simulink model "kalman_filter"  (R2020b)
settings: Solver=ode1  StartTime=0.0  StopTime=30  FixedStep=0.002  RelTol=1e-3  EnableMultiTasking=on
PreLoadFcn:
  | quanser_aero_lqr
undefined symbols (not defined in the file or in its folder): HIL, qc_get_step_size
libraries: quarc_library x4
settings Model: SimulationMode=external  ExtModeTrigDuration=20000  Creator=MLevis  LastModifiedBy=ffsandva
settings SolverCC: PositivePriorityOrder=on
settings DataIOCC: LimitDataPoints=on  SaveFormat=Array  ReturnWorkspaceOutputs=off
settings OptimizationCC: LifeSpan=inf
settings DebuggingCC: SolverPrmCheckMsg=warning  SFUnexpectedBacktrackingDiag=warning  SFNoUnconditionalDefaultTransitionDiag=warning  SFExecutionAtInitializationDiag=none  ArithmeticOperatorsInVariantConditions=warning
settings HardwareCC: ProdBitPerPointer=32  ProdBitPerSizeT=32  ProdBitPerPtrDiffT=32  ProdLargestAtomicFloat=None  ProdIntDivRoundTo=Undefined  ProdEndianess=Unspecified  ProdWordSize=32  ProdHWDeviceType=32-bit Generic
settings ModelReferenceCC: PropagateSignalLabelsOutOfModel=off
settings SFSimCC: SimUseLocalCustomCode=off  CustomCodeUndefinedFunction=UseInterfaceOnly
settings RTWCC: Description=QUARC Win64 Target  SystemTargetFile=quarc_win64.tlc  TemplateMakefile=quarc_default_tmf  RTWUseLocalCustomCode=off
settings CodeAppCC: StateflowObjectComments=on
settings STFCustomTargetCC: CPPClassGenCompliant=off
settings GRTTargetCC: TargetLangStandard=C89/C90 (ANSI)  ParMdlRefBuildCompliant=off  CompOptLevelCompliant=off  CombineOutputUpdateFcns=off  MatFileLogging=off  CPPClassGenCompliant=off  GRTInterface=on  UseToolchainInfoCompliant=off  ExtMode=on  ExtModeMexFile=quarc_comm
settings ConfigComp: CovMetricSettings=dw  CovSaveCumulativeToWorkspaceVar=on  CovSaveSingleToWorkspaceVar=on  CovExternalEMLEnable=off  CovSFcnEnable=off

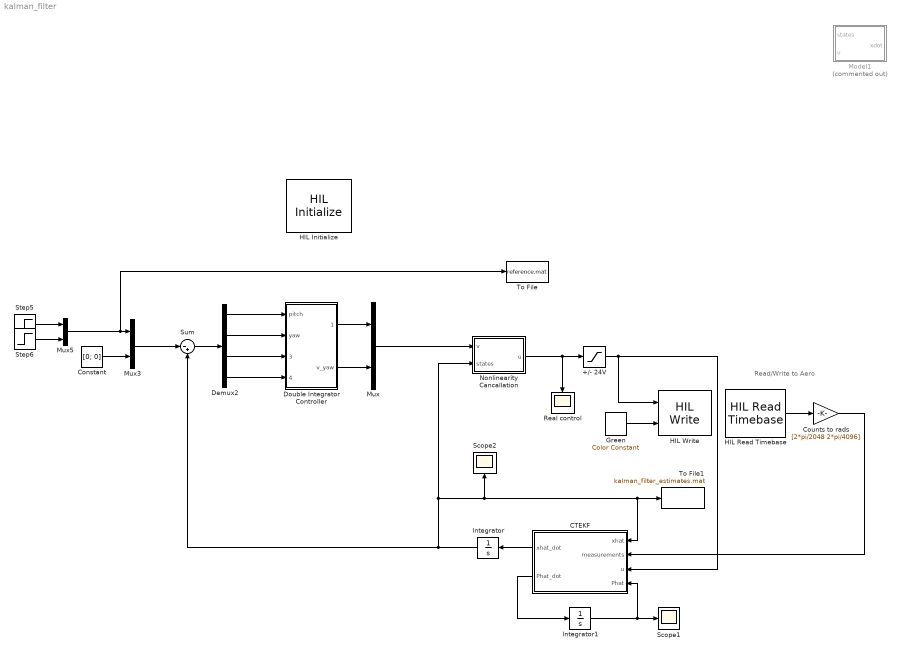
== system kalman_filter ==
  note: Read/Write to Aero
  +/- 24V : Saturate  UpperLimit=24  LowerLimit=-24
  CTEKF : MATLAB Function  TreatAsAtomicUnit=on
  Constant : Constant  Value=[0; 0]
  Counts to rads : Gain  Gain=[2*pi/2048 2*pi/4096]
  Demux2 : Demux
  Double Integrator Controller : Subsystem
  Green : quarc_library/Sources/Signals/Color Constant  color=[0 1 0]
      settings: SourceProductName=QUARC Targets
  HIL Initialize : quarc_library/Data Acquisition/Generic/Configuration/HIL Initialize  Priority=-99  object_name=HIL-1  board_type=quanser_aero_usb  board_number=0  board_options=""  exclusive=off  active=off  hardware_clocks=[0]  clock_modes=[]  initial_clock_frequencies=[]  set_clock_params_at_start=off  set_clock_params_at_switch_in=off  set_clock_frequencies_at_start=off  set_clock_frequencies_at_switch_in=off  analog_input_channels=[0:1]  analog_input_configurations=[]  analog_input_maximums=3  analog_input_minimums=-3  set_analog_input_params_at_start=off  set_analog_input_params_at_switch_in=off  analog_output_channels=[0:1]  analog_output_maximums=24  analog_output_minimums=-24  initial_analog_outputs=[0]  final_analog_outputs=[0]  watchdog_analog_outputs=[0]  set_analog_output_params_at_start=off  set_analog_output_params_at_switch_in=off  set_analog_outputs_at_start=on  set_analog_outputs_at_switch_in=off  set_analog_outputs_at_terminate=on  set_analog_outputs_at_switch_out=off  set_analog_outputs_on_watchdog=on  digital_input_channels=[]  digital_output_channels=[0:1]  digital_output_configuration=[]  initial_digital_outputs=[1]  final_digital_outputs=[0]  watchdog_digital_outputs=[0]  set_digital_output_params_at_start=off  set_digital_output_params_at_switch_in=off  set_digital_outputs_at_start=on  set_digital_outputs_at_switch_in=off  set_digital_outputs_at_terminate=on  set_digital_outputs_at_switch_out=off  set_digital_outputs_on_watchdog=on  encoder_channels=[0:3]  quadrature=[4]  encoder_filter_frequency=[]  initial_encoder_counts=[0]  set_encoder_params_at_start=off  set_encoder_params_at_switch_in=off  set_encoder_counts_at_start=on  set_encoder_counts_at_switch_in=off  pwm_channels=[]  pwm_modes=[]  pwm_frequency=[]  pwm_configuration=[]  pwm_alignment=[]  pwm_polarity=[]  pwm_leading_deadband=[]  pwm_trailing_deadband=[]  initial_pwm_outputs=[]  final_pwm_outputs=[]  watchdog_pwm_outputs=[]  set_pwm_params_at_start=off  set_pwm_params_at_switch_in=off  set_pwm_outputs_at_start=off  set_pwm_outputs_at_switch_in=off  set_pwm_outputs_at_terminate=off  set_pwm_outputs_at_switch_out=off  set_pwm_outputs_on_watchdog=off  other_output_channels=[11000:11002]  initial_other_outputs=[0 1 0]  final_other_outputs=[1 0 0]  watchdog_other_outputs=[0 0 1]  set_other_outputs_at_start=on  set_other_outputs_at_switch_in=off  set_other_outputs_at_terminate=on  set_other_outputs_at_switch_out=off  set_other_outputs_on_watchdog=on
  HIL Read Timebase : quarc_library/Data Acquisition/Generic/Timebases/HIL Read Timebase  object_name=HIL-1  clock=0  analog_channels=[0:1]  encoder_channels=[2:3]  digital_channels=[]  other_channels=[4000 4002 14000 14001]  active=on  vector_output=on  data_type_mode=Inherit via back propagation  encoder_data_type=double  digital_data_type=boolean  overflow_mode=Error on overflow  samples_in_buffer=max(ceil(1/qc_get_step_size), 1)
  HIL Write : quarc_library/Data Acquisition/Generic/Immediate I//O/HIL Write  object_name=HIL-1  analog_channels=[0:1]  pwm_channels=[]  digital_channels=[]  other_channels=[11000:11002]  sample_time=-1  active=off  vector_input=on
  Integrator : Integrator  InitialCondition=[0;0;0;0]
  Integrator1 : Integrator  InitialCondition=zeros(4)
  Model1 : MATLAB Function  Commented=on  TreatAsAtomicUnit=on
  Mux : Mux  Inputs=2
  Mux3 : Mux  Inputs=2
  Mux5 : Mux  Inputs=2
  Nonlinearity Cancallation : MATLAB Function  TreatAsAtomicUnit=on
  Real control : Scope
  Scope1 : Scope
  Scope2 : Scope
  Step5 : Step  Time=5  After=pi/6  SampleTime=0
  Step6 : Step  Time=5  After=pi/4  SampleTime=0
  Sum : Sum  Inputs=|-+
  To File : ToFile  Filename=reference.mat
  To File1 : ToFile  Filename=kalman_filter_estimates.mat  MatrixName=kalman_filter_estimates
  wires:
  HIL Read Timebase/2 -> Counts to rads/1
  +/- 24V/1 -> HIL Write/1, CTEKF/3(u)
  Green/1 -> HIL Write/2
  Double Integrator Controller/1(v_pitch) -> Mux/1
  Double Integrator Controller/2(v_yaw) -> Mux/2
  Demux2/1 -> Double Integrator Controller/1(pitch)
  Demux2/2 -> Double Integrator Controller/2(yaw)
  Demux2/3 -> Double Integrator Controller/3(pitch_dot)
  Demux2/4 -> Double Integrator Controller/4(yaw_dot)
  Sum/1 -> Demux2/1
  Mux5/1 -> To File/1, Mux3/1
  Constant/1 -> Mux3/2
  Mux3/1 -> Sum/1
  Mux/1 -> Nonlinearity Cancallation/1(v)
  Nonlinearity Cancallation/1(u) -> Real control/1, +/- 24V/1
  Step6/1 -> Mux5/2
  Step5/1 -> Mux5/1
  CTEKF/2(Phat_dot) -> Integrator1/1
  Integrator1/1 -> Scope1/1, CTEKF/4(Phat)
  CTEKF/1(xhat_dot) -> Integrator/1
  Counts to rads/1 -> CTEKF/2(measurements)
  Integrator/1 -> Nonlinearity Cancallation/2(states), To File1/1, CTEKF/1(xhat), Scope2/1, Sum/2

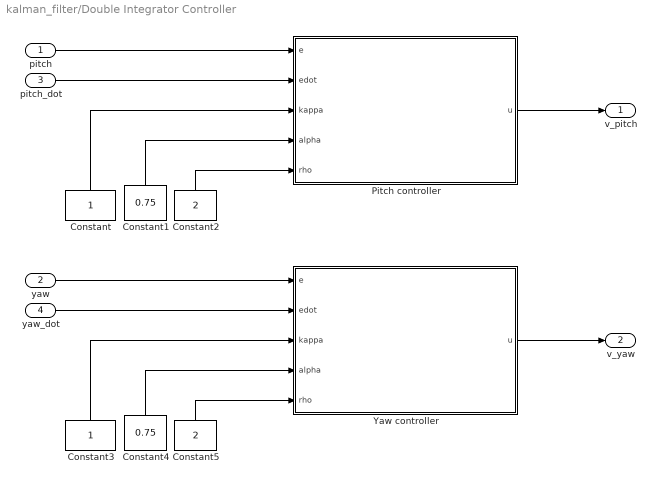
== system kalman_filter/Double Integrator Controller ==
  pitch : Inport
  yaw : Inport  Port=2
  pitch_dot : Inport  Port=3
  yaw_dot : Inport  Port=4
  Constant : Constant
  Constant1 : Constant  Value=0.75
  Constant2 : Constant  Value=2
  Constant3 : Constant
  Constant4 : Constant  Value=0.75
  Constant5 : Constant  Value=2
  Pitch controller : MATLAB Function  TreatAsAtomicUnit=on
  Yaw controller : MATLAB Function  TreatAsAtomicUnit=on
  v_pitch : Outport
  v_yaw : Outport  Port=2
  wires:
  pitch/1 -> Pitch controller/1(e)
  Constant/1 -> Pitch controller/3(kappa)
  Constant1/1 -> Pitch controller/4(alpha)
  Constant2/1 -> Pitch controller/5(rho)
  pitch_dot/1 -> Pitch controller/2(edot)
  Constant3/1 -> Yaw controller/3(kappa)
  Constant5/1 -> Yaw controller/5(rho)
  Constant4/1 -> Yaw controller/4(alpha)
  yaw/1 -> Yaw controller/1(e)
  yaw_dot/1 -> Yaw controller/2(edot)
  Yaw controller/1(u) -> v_yaw/1
  Pitch controller/1(u) -> v_pitch/1

== matlab function kalman_filter/Model1 ==
  data: states input; u input; xdot output
function xdot = QuanserAeroKumar(states, u)
    pitch = states(1);
%     yaw = states(2);
    pitch_dot = states(3);
    yaw_dot = states(4);

    g = 9.81;

    Jp = 2.15e-2;
    Jy = 2.37e-2;
    dc = 3.25e-3;
    dt = 0.158;
    mb = 1.075;
       
    Rm = 8.4;
    kt = 0.042;
    km = 0.042;
    kd = 1e-5;
    
    Kpp = 0.0011;                                                                                                                                                                                                                                                                                                                                                                                                                                                                                                                                                                                                                                                                                                                                                                                                                                                                                                                                                                                                                                                                                                                                                                                                                                                                                                                                                                                                                                                                                                                                                                                                                                                                                                                                                                                                                                                                                                                                                                                                                                                                                                                                                                                                                                                                                                                                                                                                                                                                                                                                                                                                                                                                                                                                                                                                                                                                                                                                                                                                                                                                                                                                                                                                                                                                                                                                                                                                                                                                                                                                                                                                                                                                                                                                                                                                                                                                                                                                                                                                                                                                                                                                                                                                                                                                                                                                                                                                                                                                                                                                                                                                                                                                                                                                                                                                                                                                                                                                                                                                                                                                                                                                                                                                                                                                                                                                                                                                                                                                                                                                                                                                                                                                                                                                                                                                                                                                                                                                                                                                                                                                                                                                                                                                                                                                                                                                                                                                                                                                                                                                                                                                                                                                                                                                                                                                                                                                                                                                                                                                                                                                                                                                                                                                                                                                                                                                                                                                                                                                                                                                                                                                                                                                                                                                                                                                                                                                                                                                                                                                                                                                                                                                                                                                                                                                                                                                                                                                                                                                                                                                                                                                                                                                                                                                                                                                                                                                                                                                                                                                                                                                                                                                                                                                                                                                                                                                                                                                                                                                                                                                                                                                                                                                                                                                                                                                                                                                                                                                                                                                                                                                                                                                                                                                                                                                                                                                                                                                                                                                                                                                                                              
    Kpy = 0.0021;
    Kyp = -0.0027;
    Kyy = 0.0022;
    
    Jeqp = 0.0219;
    Jeqy = 0.0220;
    Bp = 0.00711;
    By = 0.0220;
    l = 0.0071;
    m = 1.0750;
    
    a = Jeqp + m * l^2;
    b = Jeqy + m * l^2 * cos(pitch)^2;

    xdot = [
       pitch_dot;
       yaw_dot;
       (Kpp * u(1) + Kpy * u(2) - Bp * pitch_dot - m*g*l*cos(pitch) - m*l^2*sin(pitch)*cos(pitch)*yaw_dot^2)/a;
       (Kyp * u(1) + Kyy * u(2) - By * yaw_dot + 2*m*l^2*sin(pitch)*cos(pitch)*pitch_dot*yaw_dot)/b;
    ];
end

== matlab function kalman_filter/Nonlinearity Cancallation ==
  data: v input; states input; u output
function u = NonlinearityCancellation(v, states)
    theta = states(1);
    psi = states(2);
    thetadot = states(3);
    psidot = states(4);
    
    % parameters
    g = 9.81;
    dt = 0.158;
    me = 0.2;
    dx = 0.016;
    
    ry = 0.02;
    my = 0.526;
    
    mpa = 0.146;
    lt = 0.165;
    mmt = 0.089;
    mtt = 0.089;
    mtc = 0.280;
    mrod = mmt + mtt + mtc;
    
    Ibyy = 2*mpa*dt^2 + 2*me*dt^2 + me*dx^2 + 1/12*mrod*lt^2;
    Ifyzz = 1/2*my*ry^2;
    
    M = [
        Ibyy, 0;
        0, Ifyzz + Ibyy * cos(theta)^2;
    ];
    C = [
        0, Ibyy * psidot * cos(theta)*sin(theta);
        0, -2*Ibyy * thetadot * cos(theta)*sin(theta);
    ];
    gvec = [
        dx * g * me * sin(theta);
        0;
    ];

    Kmtheta = 1.26e-6;
    Kttheta = 1.08e-6;
    Kmpsi = Kttheta;
    Ktpsi = Kmtheta; 

    K_omega = 17.38;
    
    B = K_omega^2 * dt * [
        Kmtheta, Kttheta;
        -Kmpsi * cos(theta), Ktpsi * cos(theta);
    ];

    d1 = 0.0031;
    d2 = 0.0075;

    D = [
        d1, 0;
        0, d2;
    ];

    q = [
        theta;
        psi;
    ];
    qdot = [
        thetadot;
        psidot;
    ];

    utilde = B \ (M*v + C * qdot + D * qdot + gvec);
    u = sign(utilde) .* sqrt(abs(utilde));
end

== matlab function kalman_filter/Double Integrator Controller/Yaw controller ==
  data: e input; u output; edot input; kappa input; alpha input; rho input
function u = HomogeneousFiniteTimeController(e, edot, kappa, alpha, rho)
    % u = HomogeneousFiniteTimeController(e, edot, kappa, alpha, rho) computes
    % the feedback control for an orbital terminal sliding mode controller 
    % given the parameters kappa, alpha and rho.
    % See Sætre (2022) p. 56 for a derivation of the controller:
    % - https://ntnuopen.ntnu.no/ntnu-xmlui/handle/11250/3034741
    %
    % Author:   Finn F. Sandvand
    % Date:     17th Oct 2024
    % Revisions: 

    sigma = edot + kappa * sign(e) * abs(e)^alpha;
    mu = alpha * kappa^(1/alpha) + rho;
    u = alpha * kappa^2 * sign(e) * abs(e)^(2*alpha-1) ...
        - mu * sign(sigma) * abs(sigma)^((2*alpha-1)/alpha);
end

== matlab function kalman_filter/Double Integrator Controller/Pitch controller ==
  data: e input; u output; edot input; kappa input; alpha input; rho input
function u = HomogeneousFiniteTimeController(e, edot, kappa, alpha, rho)
    % u = HomogeneousFiniteTimeController(e, edot, kappa, alpha, rho) computes
    % the feedback control for an orbital terminal sliding mode controller 
    % given the parameters kappa, alpha and rho.
    % See Sætre (2022) p. 56 for a derivation of the controller:
    % - https://ntnuopen.ntnu.no/ntnu-xmlui/handle/11250/3034741
    %
    % Author:   Finn F. Sandvand
    % Date:     31th Oct 2024
    % Revisions: 

    sigma = edot + kappa * sign(e) * abs(e)^alpha;
    mu = alpha * kappa^(1/alpha) + rho;
    u = alpha * kappa^2 * sign(e) * abs(e)^(2*alpha-1) ...
        - mu * sign(sigma) * abs(sigma)^((2*alpha-1)/alpha);
end

== matlab function kalman_filter/CTEKF ==
  data: xhat input; measurements input; xhat_dot output; u input; Phat input; Phat_dot output
function [xhat_dot, Phat_dot] = ExtendedKalmanFilter(xhat, measurements, u, Phat)
    theta = xhat(1);
    psi = xhat(2);
    thetadot = xhat(3);
    psidot = xhat(4);
    
    utilde = u.^2;
    utilde1 = utilde(1);
    utilde2 = utilde(2);
    
    %R = diag([2.36e-6; 5.8974e-07]);
    R = eye(2);
    Q = diag([0; 0; 1; 1]);

    % parameters
    g = 9.81;
    dt = 0.158;
    me = 0.2;
    dx = 0.016;
    
    ry = 0.02;
    my = 0.526;
    
    mpa = 0.146;
    lt = 0.165;
    mmt = 0.089;
    mtt = 0.089;
    mtc = 0.280;
    mrod = mmt + mtt + mtc;
    
    Ibyy = 2*mpa*dt^2 + 2*me*dt^2 + me*dx^2 + 1/12*mrod*lt^2;
    Ifyzz = 1/2*my*ry^2;

%     kt = 0.042;
%     km = 0.042;
%     kd = 1e-5;
%     Rm = 8.4;
    
    % Komega = kt / (kt * km + kd * Rm);
    Komega = 17.38;
    
%     Kmtheta = 1.58e-6;
%     Kttheta = 1.35e-6;
    Kmtheta = 1.26e-6;
    Kttheta = 1.08e-6;
    Kmpsi = Kttheta;
    Ktpsi = Kmtheta; 
%     Kmpsi = 4.81e-07;
%     Ktpsi = 6.88e-07; 
    
%     d1 = 0.00711;
%     d2 = 0.0220;
    d1 = 0.0031;
    d2 = 0.0075;

    F = [
                                                                                                                                                                                                                                                                                                                                                                                           0, 0,                                                                 1,                                                              0;
                                                                                                                                                                                                                                                                                                                                                                                           0, 0,                                                                 0,                                                              1;
                                                                                                                                                                                                                                                                                                                             -(Ibyy*(2*cos(theta)^2 - 1)*psidot^2 + dx*g*me*cos(theta))/Ibyy, 0,                                                          -d1/Ibyy,                                           -psidot*sin(2*theta);
        (4*Ibyy*psidot*thetadot*(2*cos(theta)^2 - 1) + 2*Kmpsi*Komega^2*dt*utilde1*sin(theta) - 2*Komega^2*Ktpsi*dt*utilde2*sin(theta))/(Ibyy + 2*Ifyzz + Ibyy*(2*cos(theta)^2 - 1)) - (2*Ibyy*cos(theta)*sin(theta)*(d2*psidot + Kmpsi*Komega^2*dt*utilde1*cos(theta) - Komega^2*Ktpsi*dt*utilde2*cos(theta) - 2*Ibyy*psidot*thetadot*cos(theta)*sin(theta)))/(Ibyy*cos(theta)^2 + Ifyzz)^2, 0, (2*Ibyy*psidot*cos(theta)*sin(theta))/(Ibyy*cos(theta)^2 + Ifyzz), -(d2 - Ibyy*thetadot*sin(2*theta))/(Ibyy*cos(theta)^2 + Ifyzz);
    ];
    H = [eye(2), zeros(2)];
    h = H * xhat;

    M = [
        Ibyy, 0;
        0, Ifyzz + Ibyy * cos(theta)^2;
    ];
    C = [
        0, Ibyy * psidot * cos(theta)*sin(theta);
        0, -2*Ibyy * thetadot * cos(theta)*sin(theta);
    ];
    gvec = [
        dx * g * me * sin(theta);
        0;
    ];
    B = Komega^2 * dt * [
        Kmtheta, Kttheta;
        -Kmpsi * cos(theta), Ktpsi * cos(theta);
    ];
    D = [
        d1, 0;
        0, d2;
    ];
    qdot = [
        thetadot;
        psidot;
    ];
    
    f = [
        qdot;
        M \ (B*utilde - C*qdot - gvec - D*qdot);
    ];
    

    K = Phat * H' / R;
    xhat_dot = f + K * (measurements - h);
    Phat_dot = F * Phat + Phat * F' + Q - K * H * Phat;
end
